simulink model "filter_IMU0x2810x2E10x29_v2_SC"  (R2023b)
settings: Solver=FixedStepAuto  StartTime=0.0  StopTime=inf  FixedStep=Ts  RelTol=1e-3  EnableMultiTasking=on
InitFcn:
  | %Define the sampling time
  | Ts=0.003; %0.001
  | Ts2 = Ts;
  | Ts_IMU = Ts;
  | 
  | %% Low pass filter
  | %Filter coefficient (for the averaging)
  | %The averaging window is around 5*tau
  | T=0.1; %0.1
  | 
  | %The constant alpha is used just to avoid more calculations
  | alpha = (T/Ts)/(1+T/Ts);
libraries: simulink_extras x2, bbblueSensorLib x1
settings Model: SimulationMode=external  ExtModeTrigDuration=100  Creator=kknud  LastModifiedBy=kknud
settings SolverCC: PositivePriorityOrder=on
settings OptimizationCC: EnhancedBackFolding=on  PassReuseOutputArgsAs=Individual arguments  ZeroExternalMemoryAtStartup=off  ZeroInternalMemoryAtStartup=off  MaxStackSize=64  OptimizeBlockOrder=speed  DifferentSizesBufferReuse=on  OptimizationCustomize=off  EfficientTunableParamExpr=on
settings DebuggingCC: ParameterTunabilityLossMsg=error
settings HardwareCC: ProdBitPerPointer=32  ProdBitPerSizeT=32  ProdBitPerPtrDiffT=32  ProdLargestAtomicInteger=Long  ProdLargestAtomicFloat=Double  ProdWordSize=32  ProdHWDeviceType=ARM Compatible->ARM Cortex
settings SFSimCC: MATLABDynamicMemAlloc=off
settings RTWCC: Description=Embedded Coder  SystemTargetFile=ert.tlc  HardwareBoard=BeagleBone Blue  TLCOptions="-aInlineSetEventsForThisBaseRateFcn=TLC_FALSE -aSuppressMultiTaskScheduler=TLC_FALSE  -aRateBasedStepFcn=0"  TemplateMakefile=ert_default_tmf  Toolchain=GNU GCC BeagleBone Blue  BuildConfiguration=Faster Runs
settings CodeAppCC: ForceParamTrailComments=on  IgnoreCustomStorageClasses=off  OperatorAnnotations=on  SimulinkDataObjDesc=on  SFDataObjDesc=on  InsertBlockDesc=on
settings ERTTargetCC: SupportContinuousTime=on  SupportVariableSizeSignals=on  ExtMode=on  ExtModeMexArgs='192.168.7.2' 0 17725

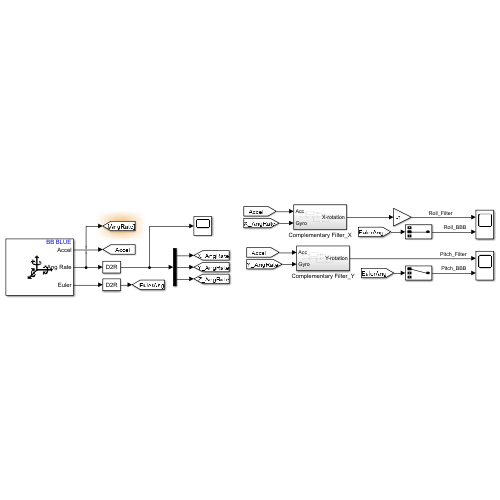
[thumbnail: Simulink's stored preview of the top-level diagram]
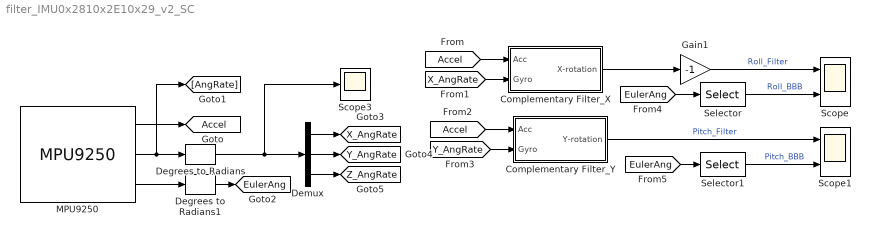
== system filter_IMU0x2810x2E10x29_v2_SC ==
  Complementary Filter_X : Subsystem
  Complementary Filter_Y : Subsystem
  Degrees to Radians : simulink_extras/Transformations/Degrees to Radians
  Degrees to Radians1 : simulink_extras/Transformations/Degrees to Radians
  Demux : Demux  Outputs=3
  Gain1 : Gain  Gain=-1
  MPU9250 : bbblueSensorLib/MPU9250  OperationMode=DMP  Accel=on  AngularRate=on  Ak8963Field=off  EulerAngles=on  Quat=off  AccelRange=2G  Acceldlpf=1  GyroRange=250 dps  Gyrodlpf=1  DmpOdr=200 Hz  SampleTime=0.003
  Scope : Scope  NumInputPorts=2
  Scope1 : Scope  NumInputPorts=2
  Scope3 : Scope
  Selector : Selector  InputPortWidth=3  IndexOptions=Index vector (dialog)  Indices=[2]  OutputSizes=1
  Selector1 : Selector  InputPortWidth=3  IndexOptions=Index vector (dialog)  Indices=[1]  OutputSizes=1
  tag scope: Accel=global, EulerAng=global, X_AngRate=global, Y_AngRate=global, Z_AngRate=global
  wires:
  Complementary Filter_X/1(X-rotation) -> Gain1/1
  MPU9250/1 -> [Accel]
  [Accel] -> Complementary Filter_X/1(Acc)
  [X_AngRate] -> Complementary Filter_X/2(Gyro)
  [Y_AngRate] -> Complementary Filter_Y/2(Gyro)
  [Accel] -> Complementary Filter_Y/1(Acc)
  Complementary Filter_Y/1(Y-rotation) -> Scope1/1  "Pitch_Filter"
  Selector/1 -> Scope/2  "Roll_BBB"
  [EulerAng] -> Selector/1
  Selector1/1 -> Scope1/2  "Pitch_BBB"
  [EulerAng] -> Selector1/1
  MPU9250/3 -> Degrees to Radians1/1
  Demux/1 -> [X_AngRate]
  Demux/2 -> [Y_AngRate]
  Demux/3 -> [Z_AngRate]
  Degrees to Radians/1 -> Demux/1, Scope3/1
  MPU9250/2 -> [AngRate], Degrees to Radians/1
  Degrees to Radians1/1 -> [EulerAng]
  Gain1/1 -> Scope/1  "Roll_Filter"

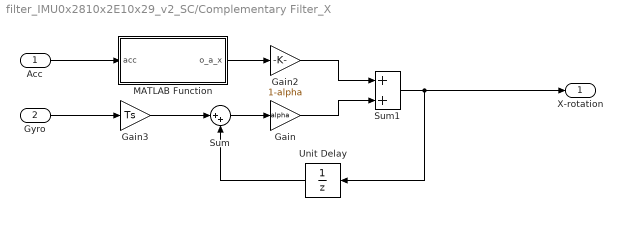
== system filter_IMU0x2810x2E10x29_v2_SC/Complementary Filter_X ==
  Acc : Inport
  Gyro : Inport  Port=2
  Gain : Gain  Gain=alpha
  Gain2 : Gain  Gain=1-alpha
  Gain3 : Gain  Gain=Ts
  MATLAB Function : MATLAB Function  TreatAsAtomicUnit=on
  Sum : Sum  Inputs=|++
  Sum1 : Sum
  Unit Delay : UnitDelay  SampleTime=-1  HasFrameUpgradeWarning=on
  X-rotation : Outport
  wires:
  MATLAB Function/1(o_a_x) -> Gain2/1
  Gain/1 -> Sum1/2
  Sum/1 -> Gain/1
  Acc/1 -> MATLAB Function/1(acc)
  Gain2/1 -> Sum1/1
  Unit Delay/1 -> Sum/2
  Gain3/1 -> Sum/1
  Gyro/1 -> Gain3/1
  Sum1/1 -> X-rotation/1, Unit Delay/1

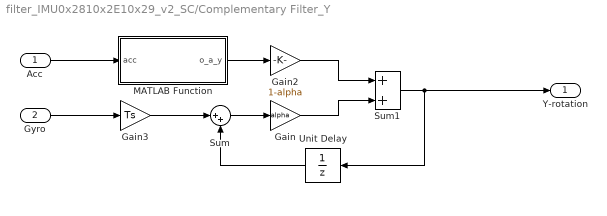
== system filter_IMU0x2810x2E10x29_v2_SC/Complementary Filter_Y ==
  Acc : Inport
  Gyro : Inport  Port=2
  Gain : Gain  Gain=alpha
  Gain2 : Gain  Gain=1-alpha
  Gain3 : Gain  Gain=Ts
  MATLAB Function : MATLAB Function  TreatAsAtomicUnit=on
  Sum : Sum  Inputs=|++
  Sum1 : Sum
  Unit Delay : UnitDelay  SampleTime=-1  HasFrameUpgradeWarning=on
  Y-rotation : Outport
  wires:
  MATLAB Function/1(o_a_y) -> Gain2/1
  Gain/1 -> Sum1/2
  Sum/1 -> Gain/1
  Acc/1 -> MATLAB Function/1(acc)
  Gain2/1 -> Sum1/1
  Unit Delay/1 -> Sum/2
  Gain3/1 -> Sum/1
  Gyro/1 -> Gain3/1
  Sum1/1 -> Y-rotation/1, Unit Delay/1

== matlab function filter_IMU0x2810x2E10x29_v2_SC/Complementary Filter_X/MATLAB Function ==
  data: acc input; o_a_x output
function o_a_x = fcn(acc)

acc_x = acc(1);
acc_z = acc(3);

o_a_x = atan(acc_x/acc_z);

end

== matlab function filter_IMU0x2810x2E10x29_v2_SC/Complementary Filter_Y/MATLAB Function ==
  data: acc input; o_a_y output
function o_a_y = fcn(acc)

acc_y = acc(2);
acc_z = acc(3);

o_a_y = atan(acc_y/acc_z);

end
